simulink model "PROBLEM8"  (R2020b)
settings: Solver=VariableStepAuto  StartTime=0.0  StopTime=10.0  RelTol=1e-3
settings Model: Creator=ARPITA  LastModifiedBy=ARPITA

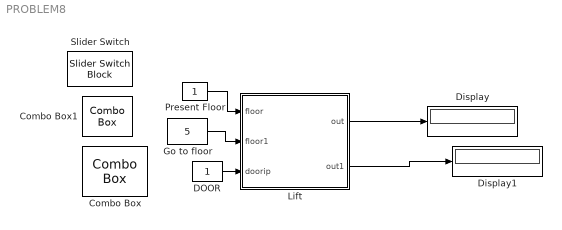
== system PROBLEM8 ==
  Combo Box : ComboBox  SelectedLabel=FLOOR4
      settings: Values={{'GROUND', 'FLOOR1', 'FLOOR2', 'FLOOR3', 'FLOOR4'}, [1 2 3 4 5]}
  Combo Box1 : ComboBox  SelectedLabel=GROUND
      settings: Values={{'GROUND', 'FLOOR1', 'FLOOR2', 'FLOOR3', 'FLOOR4'}, [1 2 3 4 5]}
  DOOR : Constant
  Display : Display
  Display1 : Display
  Go to floor : Constant  Value=5
  Lift : Stateflow chart  TreatAsAtomicUnit=on
  Present Floor : Constant
  Slider Switch : SliderSwitchBlock
      settings: Values={{'Off', 'On'}, [0 1]}
  wires:
  Lift/1(out) -> Display/1
  Present Floor/1 -> Lift/1(floor)
  Lift/2(out1) -> Display1/1
  DOOR/1 -> Lift/3(doorip)
  Go to floor/1 -> Lift/2(floor1)

== stateflow chart PROBLEM8/Lift ==
  state Door_open
    (history)
    state Lift_For_five_floor
      (history)
      state Floor1
        entry:
        present=1;
        out=1;
      state Floor2
        entry:
        out=2;
        present=out;
      state Floor3
        entry:
        out=3;
        present=out;
      state Floor4
        entry:
        out=4;
        present=out;
      state Floor5
        entry:
        out=5;
        present=out
      Door_open.Lift_For_five_floor.Floor1 -> Door_open.Lift_For_five_floor.Floor1 [order 2] : [present==floor]
      (default) -> Door_open.Lift_For_five_floor.Floor1
      Door_open.Lift_For_five_floor.Floor3 -> Door_open.Lift_For_five_floor.Floor4 [order 1] : [present<floor]
      Door_open.Lift_For_five_floor.Floor2 -> Door_open.Lift_For_five_floor.Floor3 [order 1] : [present<floor]
      Door_open.Lift_For_five_floor.Floor4 -> Door_open.Lift_For_five_floor.Floor5 [order 1] : [present<floor]
      Door_open.Lift_For_five_floor.Floor1 -> Door_open.Lift_For_five_floor.Floor2 [order 1] : [present<floor]
      Door_open.Lift_For_five_floor.Floor5 -> Door_open.Lift_For_five_floor.Floor5 [order 2] : [floor==present]
      Door_open.Lift_For_five_floor.Floor5 -> Door_open.Lift_For_five_floor.Floor4 [order 1] : [present>floor]
      Door_open.Lift_For_five_floor.Floor4 -> Door_open.Lift_For_five_floor.Floor3 [order 2] : [present>floor]
      Door_open.Lift_For_five_floor.Floor2 -> Door_open.Lift_For_five_floor.Floor1 [order 2] : [present>floor]
      Door_open.Lift_For_five_floor.Floor3 -> Door_open.Lift_For_five_floor.Floor2 [order 2] : [present>floor]
    state Second_input
      (history)
      state Floor1
        entry:
        present=1;
        out1=1;
      state Floor2
        entry:
        out1=2;
        present=out1;
      state Floor3
        entry:
        out1=3;
        present=out1;
      state Floor4
        entry:
        out1=4;
        present=out1;
      state Floor5
        entry:
        out1=5;
        present=out1;
      Door_open.Second_input.Floor1 -> Door_open.Second_input.Floor1 [order 2] : [present==floor1]
      (default) -> Door_open.Second_input.Floor1
      Door_open.Second_input.Floor3 -> Door_open.Second_input.Floor4 [order 1] : [present<floor1]
      Door_open.Second_input.Floor2 -> Door_open.Second_input.Floor3 [order 1] : [present<floor1]
      Door_open.Second_input.Floor4 -> Door_open.Second_input.Floor5 [order 1] : [present<floor1]
      Door_open.Second_input.Floor1 -> Door_open.Second_input.Floor2 [order 1] : [present<floor1]
      Door_open.Second_input.Floor5 -> Door_open.Second_input.Floor5 [order 2] : [floor==present]
      Door_open.Second_input.Floor5 -> Door_open.Second_input.Floor4 [order 1] : [present>floor1]
      Door_open.Second_input.Floor4 -> Door_open.Second_input.Floor3 [order 2] : [present>floor1]
      Door_open.Second_input.Floor2 -> Door_open.Second_input.Floor1 [order 2] : [present>floor1]
      Door_open.Second_input.Floor3 -> Door_open.Second_input.Floor2 [order 2] : [present>floor1]
    (default) -> Lift_For_five_floor
    Lift_For_five_floor -> Second_input : [present==floor]
  state Door_close
    entry:
    out=floor;
    out1=0;
    (history)
  (default) -> Door_close
  Door_open -> Door_close : [doorip==1]
  Door_close -> Door_open : [doorip==0]
  data: floor input; present local; out output; floor1 input; out1 output; doorip input
